simulink model "vsi_avg_zdc_v01_Ph2N"  (Simulink 7.7)
settings: Solver=ode45  StartTime=0.0  StopTime=0.5  MaxStep=25e-6  RelTol=1e-4  AbsTol=1e-5
values from neighbouring files (symbols this model uses):
  C = 21.308e-6    (= 2.1308e-05)    [Current_Loop_Design.m]    (also in VSI_Controller_Design.m = 3.13e-05; VSI_TFs_i_loop.m = 2.2e-05; VSI_TFs_o_loop.m = 4.13e-05; VSI_TFs_v_loop.m = 4.1308e-05)
  L = (0.75879e-3)/(2/3)    (= 0.001138185)    [Current_Loop_Design.m]    (also in VSI_Controller_Design.m = 0.0011; VSI_TFs_i_loop.m = 0.0012; VSI_TFs_o_loop.m = 0.0011; VSI_TFs_v_loop.m = 0.0011)
  R = 15    [Current_Loop_Design.m]    (also in ZVSI_il_tf_cal_sim_comp_frd_model_v1.m; ZVSI_ol_tf_cal_sim_comp_frd_model_v1.m; ZVSI_vil_tf_cal_frd_model_Monte_Carlo.m = R_rec(i); ZVSI_vil_tf_cal_sim_comp_frd_model_v1.m = 12)
  RL = 80e-3    (= 0.08)    [Current_Loop_Design.m]    (also in ZVSI_il_tf_cal_sim_comp_frd_model_v1.m = 0.15; ZVSI_ol_tf_cal_sim_comp_frd_model_v1.m = 1.5e-05; ZVSI_vil_tf_cal_frd_model_Monte_Carlo.m = 0.13; ZVSI_vil_tf_cal_sim_comp_frd_model_v1.m = 0.13)
  Vdc = 270    [Current_Loop_Design.m]    (also in VSI_Controller_Design.m; VSI_TFs_i_loop.m; VSI_TFs_o_loop.m; VSI_TFs_v_loop.m)
  w = 2*pi*fline    (= 2513.27412287)    [Current_Loop_Design.m]    (also in ZVSI_il_tf_cal_sim_comp_frd_model_v1.m = 15791.3670417; ZVSI_ol_tf_cal_sim_comp_frd_model_v1.m = 15791.3670417; ZVSI_vil_tf_cal_frd_model_Monte_Carlo.m = 15791.3670417; ZVSI_vil_tf_cal_sim_comp_frd_model_v1.m = 15791.3670417)
libraries: powerlib x26
settings Model: Creator=marko  LastModifiedBy=Bo  BufferReuse=off
settings OptimizationCC: BlockReduction=off  InlineParams=on  BufferReuse=off
settings DebuggingCC: AlgebraicLoopMsg=none  SolverPrmCheckMsg=none  UnconnectedInputMsg=none  UnconnectedOutputMsg=none  UnconnectedLineMsg=none  StrictBusMsg=Warning

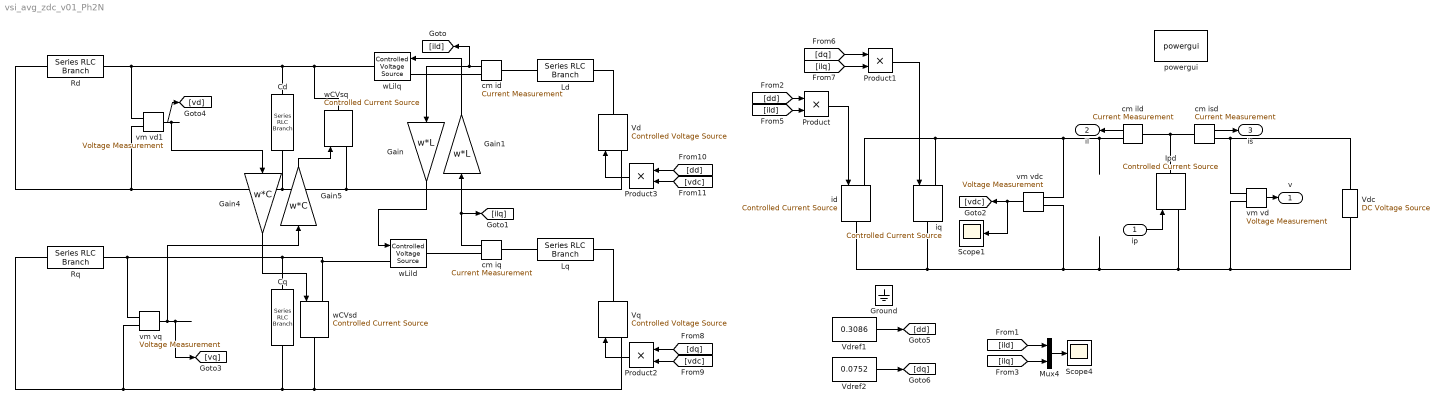
== system vsi_avg_zdc_v01_Ph2N ==
  ip : Inport
  Cd : powerlib/Elements/Series RLC Branch  PhysicalDomain=powersysdomain  SubClassName=unknown  LeftPortType=p1  RightPortType=p1  LConnTagsString=__new0  RConnTagsString=__new0  BranchType=C  Resistance=1  Inductance=1e-3  SetiL0=off  InitialCurrent=0  Capacitance=C  Setx0=off  InitialVoltage=0  Measurements=None
  Cq : powerlib/Elements/Series RLC Branch  PhysicalDomain=powersysdomain  SubClassName=unknown  LeftPortType=p1  RightPortType=p1  LConnTagsString=__new0  RConnTagsString=__new0  BranchType=C  Resistance=1  Inductance=1e-3  SetiL0=off  InitialCurrent=0  Capacitance=C  Setx0=off  InitialVoltage=0  Measurements=None
  Gain : Gain  Gain=w*L
  Gain1 : Gain  Gain=w*L
  Gain4 : Gain  Gain=w*C
  Gain5 : Gain  Gain=w*C
  Ground : powerlib/Elements/Ground  PhysicalDomain=powersysdomain  SubClassName=unknown  LeftPortType=p1  RightPortType=p1  LConnTagsString=a
  Ipd : powerlib/Electrical Sources/Controlled Current Source  SystemSampleTime=-1  Initialize=on  Source_Type=AC  Amplitude=0  Phase=0  Frequency=0  Measurements=None
  Ld : powerlib/Elements/Series RLC Branch  PhysicalDomain=powersysdomain  SubClassName=unknown  LeftPortType=p1  RightPortType=p1  LConnTagsString=__new0  RConnTagsString=__new0  BranchType=RL  Resistance=RL  Inductance=L  SetiL0=off  InitialCurrent=0  Capacitance=1e-6  Setx0=off  InitialVoltage=0  Measurements=None
  Lq : powerlib/Elements/Series RLC Branch  PhysicalDomain=powersysdomain  SubClassName=unknown  LeftPortType=p1  RightPortType=p1  LConnTagsString=__new0  RConnTagsString=__new0  BranchType=RL  Resistance=RL  Inductance=L  SetiL0=off  InitialCurrent=0  Capacitance=1e-6  Setx0=off  InitialVoltage=0  Measurements=None
  Mux4 : Mux  Inputs=2
  Product{,1..3} (4 alike) : Product  RndMeth=Zero
  Rd : powerlib/Elements/Series RLC Branch  PhysicalDomain=powersysdomain  SubClassName=unknown  LeftPortType=p1  RightPortType=p1  LConnTagsString=__new0  RConnTagsString=__new0  BranchType=R  Resistance=R  Inductance=1e-3  SetiL0=off  InitialCurrent=0  Capacitance=1e-6  Setx0=off  InitialVoltage=0  Measurements=None
  Rq : powerlib/Elements/Series RLC Branch  PhysicalDomain=powersysdomain  SubClassName=unknown  LeftPortType=p1  RightPortType=p1  LConnTagsString=__new0  RConnTagsString=__new0  BranchType=R  Resistance=R  Inductance=1e-3  SetiL0=off  InitialCurrent=0  Capacitance=1e-6  Setx0=off  InitialVoltage=0  Measurements=None
  Scope1 : Scope
      settings: YMin=264.5  YMax=275.5  SaveName=ildq_matlab  DataFormat=Array
  Scope4 : Scope
      settings: YMin=-0.25  YMax=5.25  SaveName=ildq_matlab1  DataFormat=Array
  Vd : powerlib/Electrical Sources/Controlled Voltage Source  SystemSampleTime=-1  Initialize=on  Source_Type=DC  Amplitude=0  Phase=0  Frequency=0  Measurements=None
  Vdc : powerlib/Electrical Sources/DC Voltage Source  SystemSampleTime=-1  Amplitude=Vdc  Measurements=None
  Vdref1 : Constant  Value=0.3086
  Vdref2 : Constant  Value=0.0752
  Vq : powerlib/Electrical Sources/Controlled Voltage Source  SystemSampleTime=-1  Initialize=on  Source_Type=DC  Amplitude=0  Phase=0  Frequency=0  Measurements=None
  cm id : powerlib/Measurements/Current Measurement  SystemSampleTime=-1  PhasorSimulation=off  OutputType=Complex  PSBequivalent=0
  cm ild : powerlib/Measurements/Current Measurement  SystemSampleTime=-1  PhasorSimulation=off  OutputType=Complex  PSBequivalent=0
  cm iq : powerlib/Measurements/Current Measurement  SystemSampleTime=-1  PhasorSimulation=off  OutputType=Complex  PSBequivalent=0
  cm isd : powerlib/Measurements/Current Measurement  SystemSampleTime=-1  PhasorSimulation=off  OutputType=Complex  PSBequivalent=0
  id : powerlib/Electrical Sources/Controlled Current Source  SystemSampleTime=-1  Initialize=on  Source_Type=DC  Amplitude=0  Phase=0  Frequency=0  Measurements=None
  iq : powerlib/Electrical Sources/Controlled Current Source  SystemSampleTime=-1  Initialize=on  Source_Type=DC  Amplitude=0  Phase=0  Frequency=0  Measurements=None
  powergui : powerlib/powergui  Priority=1  SystemSampleTime=-1  SimulationMode=Continuous  SampleTime=50e-6  frequency=60  SPID=off  DisableSnubberDevices=off  DisableRonSwitches=off  DisableVfSwitches=off  SwTol=0  Interpol=off  DisplayEquations=off  FunctionMessages=off  frequencyindice=0  Pbase=100e6  ErrMax=1e-4  Iterations=50  UnitsV=kV  UnitsW=MW  echomessages=off  HookPort=off  EnableUseOfTLC=off  x0status=blocks  RestoreLinks=warning  ResistiveCurrentMeasurement=off  Frange=[0:2:500]  Ylog=off  Xlog=on  ShowGrid=off  save=off  variable=ZData  ZoomFFT=on  StartTime=0.0  cycles=1  DisplayStyle=1  fundamental=60  FreqAxis=off  MaxFrequency=1000  frequencyindicesteady=1  RmsSteady=1  display=off  Ts=0  methode=off
  vm vd : powerlib/Measurements/Voltage Measurement  SystemSampleTime=-1  PhasorSimulation=off  OutputType=Complex  PSBequivalent=0
  vm vd1 : powerlib/Measurements/Voltage Measurement  SystemSampleTime=-1  PhasorSimulation=off  OutputType=Complex  PSBequivalent=0
  vm vdc : powerlib/Measurements/Voltage Measurement  SystemSampleTime=-1  PhasorSimulation=off  OutputType=Complex  PSBequivalent=0
  vm vq : powerlib/Measurements/Voltage Measurement  SystemSampleTime=-1  PhasorSimulation=off  OutputType=Complex  PSBequivalent=0
  wCVsd : powerlib/Electrical Sources/Controlled Current Source  SystemSampleTime=-1  Initialize=on  Source_Type=DC  Amplitude=0  Phase=0  Frequency=0  Measurements=None
  wCVsq : powerlib/Electrical Sources/Controlled Current Source  SystemSampleTime=-1  Initialize=on  Source_Type=DC  Amplitude=0  Phase=0  Frequency=0  Measurements=None
  wLild : powerlib/Electrical Sources/Controlled Voltage Source  SystemSampleTime=-1  Initialize=on  Source_Type=DC  Amplitude=0  Phase=0  Frequency=0  Measurements=None
  wLilq : powerlib/Electrical Sources/Controlled Voltage Source  SystemSampleTime=-1  Initialize=on  Source_Type=DC  Amplitude=0  Phase=0  Frequency=0  Measurements=None
  v : Outport
  il : Outport  Port=2
  is : Outport  Port=3
  wires:
  [ild] -> Mux4/1
  [ilq] -> Mux4/2
  Mux4/1 -> Scope4/1
  Product/1 -> id/1
  [dd] -> Product/1
  [ild] -> Product/2
  Product1/1 -> iq/1
  [dq] -> Product1/1
  [ilq] -> Product1/2
  vm vdc/1 -> [vdc], Scope1/1
  ip/1 -> Ipd/1
  vm vd/1 -> v/1
  cm ild/1 -> il/1
  cm isd/1 -> is/1
  Vdref1/1 -> [dd]
  Vdref2/1 -> [dq]
  [dq] -> Product2/1
  [vdc] -> Product2/2
  Product2/1 -> Vq/1
  [dd] -> Product3/1
  [vdc] -> Product3/2
  Product3/1 -> Vd/1
  vm vd1/1 -> [vd], Gain4/1
  vm vq/1 -> Gain5/1, [vq]
  cm iq/1 -> Gain1/1, [ilq]
  Gain1/1 -> wLilq/1
  cm id/1 -> Gain/1, [ild]
  Gain/1 -> wLild/1
  Gain4/1 -> wCVsd/1
  Gain5/1 -> wCVsq/1
  connections:
  cm ild/RConn1 -- iq/LConn1 -- id/LConn1 -- vm vdc/LConn1
  cm isd/LConn1 -- cm ild/LConn1 -- Ipd/RConn1
  Vdc/RConn1 -- cm isd/RConn1 -- vm vd/LConn1
  Vdc/LConn1 -- iq/RConn1 -- id/RConn1 -- vm vdc/LConn2 -- Ipd/LConn1 -- vm vd/LConn2
  Rq/LConn1 -- vm vq/LConn2 -- Vq/LConn1 -- wCVsd/RConn1 -- Cq/RConn1
  Rd/LConn1 -- vm vd1/LConn2 -- Vd/LConn1 -- wCVsq/LConn1 -- Cd/RConn1
  Rd/RConn1 -- wCVsq/RConn1 -- wLilq/RConn1 -- Cd/LConn1 -- vm vd1/LConn1
  Rq/RConn1 -- Cq/LConn1 -- wCVsd/LConn1 -- wLild/LConn1 -- vm vq/LConn1
  Lq/RConn1 -- Vq/RConn1
  Ld/RConn1 -- Vd/RConn1
  cm id/LConn1 -- Ld/LConn1
  cm iq/LConn1 -- Lq/LConn1
  wLild/RConn1 -- cm iq/RConn1
  wLilq/LConn1 -- cm id/RConn1
